simulink model "TwoOneTwo_allBlock"  (R2022b)
settings: Solver=VariableStepAuto  StartTime=0.0  StopTime=10.0  RelTol=1e-3
settings Model: Creator=yeyi5  LastModifiedBy=yeyi5

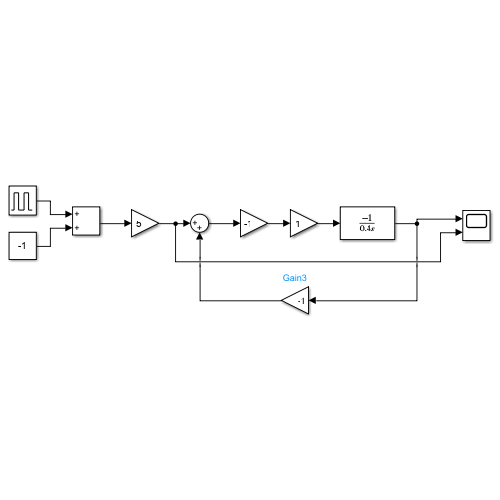
[thumbnail: Simulink's stored preview of the top-level diagram]
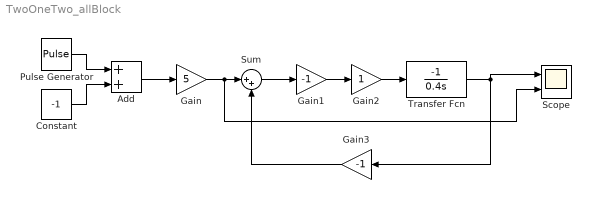
== system TwoOneTwo_allBlock ==
  Add : Sum
  Constant : Constant  Value=-1
  Gain : Gain  Gain=5
  Gain1 : Gain  Gain=-1
  Gain2 : Gain
  Gain3 : Gain  Gain=-1
  Pulse Generator : DiscretePulseGenerator  PulseType=Time based  Amplitude=2  Period=1/0.1  PulseWidth=50
  Scope : Scope  NumInputPorts=2
  Sum : Sum  Inputs=|++
  Transfer Fcn : TransferFcn  Numerator=[-1]  Denominator=[0.4 0]
  wires:
  Pulse Generator/1 -> Add/1
  Constant/1 -> Add/2
  Add/1 -> Gain/1
  Gain/1 -> Scope/2, Sum/1
  Sum/1 -> Gain1/1
  Gain1/1 -> Gain2/1
  Gain2/1 -> Transfer Fcn/1
  Gain3/1 -> Sum/2
  Transfer Fcn/1 -> Scope/1, Gain3/1
